simulink library "EngineModelsLibrary"  (R2014b)
settings: Solver=ode45  StartTime=0.0  StopTime=10.0  RelTol=1e-3
values from neighbouring files (symbols this model uses):
  k = 0.2    [ES_Run.m]    (also in ES_Run_v2.m = 10)
undefined symbols (not defined in the file or in its folder): b, COBRA_Compressor, cp, CPT_COBRA_LIB, D, etalim, gam, Newton, Pa, PARAM, Pl, pref, Ps, R, Raphson, rlim, T_0, Tref, Wclim
undefined symbols (not defined in the file): cr, e, etagain, fit_pars, kL, kS, par
(part 1 of 3)
settings Model: Creator=Mike  LastModifiedBy=rsalehi

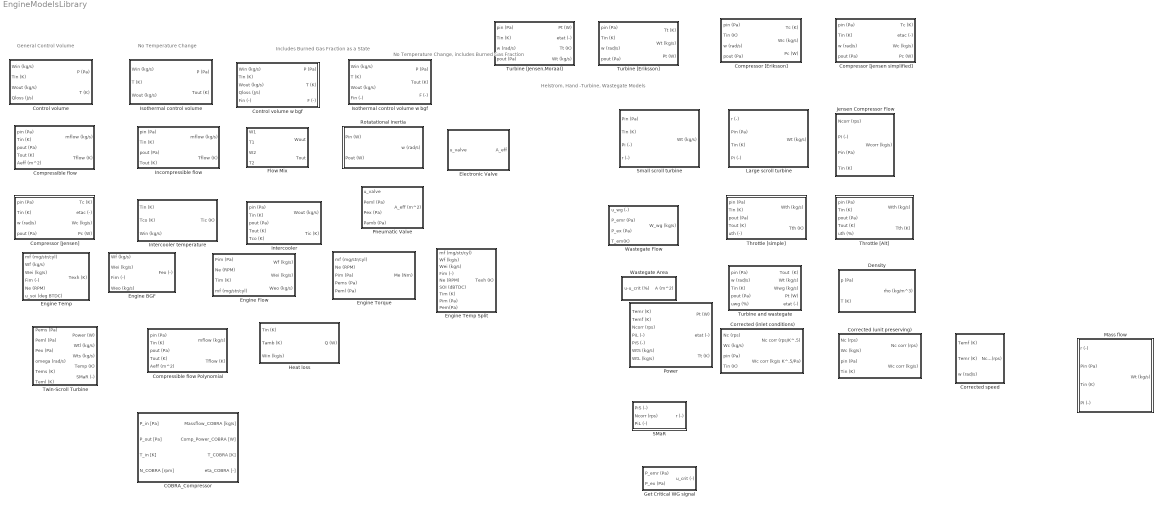
== system EngineModelsLibrary ==
  note: Helstrom, Hand -Turbine, Wastegate Models
  note: No Temperature Change, includes Burned Gas Fraction
  note: Includes Burned Gas Fraction as a State
  note: No Temperature Change
  note: General Control Volume
  COBRA_Compressor : Subsystem  Tag=Version 2 Compressor model with lookup option for efficiency  AncestorBlock=CPT_COBRA_LIB/COBRA_Compressor  mask(Controlled Power Technologies Ltd){CompWheel=C80}
      mask prompts: CompWheel "Compressor Wheel"
      mask help:
      | Basic model of COBRA electric supercharger compressor
      |
      | INPUTS:
      |
      | P_in - Gas pressure upstream of the compressor [Pa]
      | P_out - Gas pressure downstream of the compressor [Pa]
      | T_in - Gas temperature upstream of the compressor [K]
      | N_COBRA - Compressor rotational speed [rpm]
      |
      | OUTPUTS:
      |
      | Massflow_COBRA - Gas mass flow through the compressor [kg/s]
      | Comp_Power_COBRA - Power consumed by the compressor due to aerodynamic load [W]
      | T_COBRA - Gas temperature at compressor outlet [K]
      | eta_COBRA - Compressor efficiency [-]
      |
      | Use the menu selector below to choose either the C70 or C80 compressor wheels
      |
      | For further information click help or consult documentation
      mask init:
      | try 
      | load('COBRA_Compressor_Pars.mat');
      | 
      | Wheel=get_param(gcb,'CompWheel');
      | if strcmp(Wheel,'C70')==1
      |     COBRACompressor.mdotcMap=COBRACompressor.mdotcMapC70;
      |     COBRACompressor.EtaMap=COBRACompressor.EtaMapC70;
      |     COBRACompressor.max_mdotc=COBRACompressor.max_mdotc_C70;
      |     disp('C70 Wheel selected');
      | else
      |     COBRACompressor.mdotcMap=COBRACompressor.mdotcMapC80;
      |     COBRACompressor.EtaMap=COBRACompressor.EtaMapC80;
      |     COBRACompressor.max_mdotc=COBRACompressor.max_mdotc_C80;
      |     disp('C80 Wheel selected');
      | end
      | 
      | catch InitErr
      |     disp('ERROR: COBRA_Compressor_Pars.mat file must be located in same directory as model or in a directory on the Matlab path')
      | end
      mask Help:
      | COBRA Compressor Model
      | 
      | Model Description
      | 
      | The COBRA compressor model comprises a simplified lookup table implementation of the compressor maps. Taking inputs of upstream temperature and pressure, downstream pressure and compressor rotational speed, it will calculate the compressor mass airflow, required shaft power, outlet gas temperature and overall compressor isentropic efficiency. The model is designed to be used in mean value simulations and needs to be connected to plenums / volumes either side of it to function correctly.
      | 
      | Model requirements, installation and usage notes
      | 
      | The model has been created using MATLAB / Simulink Release 2014b. To use the model it should be dragged and dropped into another the Simulink model. The parameter file <COBRA_Compressor_Pars.mat> must be located in the current working directory or in a directory on the Matlab path, it is automatically loaded when the model initialises.
      | 
      | The model acts as a flow restriction element within a full simulation of the engine gas path, it requires volumes or plenums to be connected both directly upstream and downstream of it in order to provide the input and output conditions required to calculate the mass flow. The resultant mass flow must be connected both as flow into the downstream volume and flow out of the upstream volume.
      | 
      | Normally the COBRA system is used with a bypass which can be either active or passive, this has not been provided in this model but can easily be created, consult the documentation for further details.
      | 
      | No electrical or mechanical dynamics have been included in this model. For an approximation of transient response, a 1st order lag can be placed in front of the speed input to COBRA with a T90 time of approx. 300ms.
      | 
      | The option to use 2 different compressor sizes is built-in to the model. Either the C70 or C80 wheels can be chosen from a menu within the block mask, double click on the block to access this menu.
      mask TypeOptions CompWheel: C70 | C80
      mask Display:
      | mytext=get_param(gcb,'CompWheel');
      | disp(strcat(mytext,'\n'));
      | disp('Compressor');
      | %text(40,17,'Controlled Power');
      | %text(40,5,'Technologies Ltd');
  Compressible flow : Subsystem  mask{gam=1.27, R=286, PIlin=.99}
      mask prompts: gam "Specific heat ratio (-)"; R "Ideal gas constant (J/kg/K)"; PIlin "Linear segment minimum pressure ratio (-)"
      mask help: Compressible flow, see App. C in Heywood (1988). Modified by adding a linear segment for pressure ratios larger than the parameter PIlin. In this way, it is possible to avoid infinite derivative for pressure ratios close to one. -- erikhe@umich
  Compressible flow Polynomial : Subsystem  mask{gam=1.27, R=286, P=fit_pars.egr.psi}
      mask prompts: gam "Specific heat ratio (-)"; R "Ideal gas constant (J/kg/K)"; P "Psi Polynomail [3 pars]"
      mask help: Compressible flow, see App. C in Heywood (1988). Modified by adding a linear segment for pressure ratios larger than the parameter PIlin. In this way, it is possible to avoid infinite derivative for pressure ratios close to one. -- erikhe@umich
  Compressor [Eriksson] : Subsystem  mask{gam=PARAM.air.gamma, cp=PARAM.air.cp, R=PARAM.air.R, D=PARAM.compressor.D, a1=PARAM.compressor.a1, a2=PARAM.compressor.a2, pref=PARAM.compressor.pref, Tref=PARAM.compressor.Tref, Phimax=PARAM.compressor.Phimax, Ncorrmax=PARAM.compressor.Ncorrmax, etamax=PARAM.compressor.etamax, etamin=PARAM.compressor.etamin, Q=PARAM.compressor.Q}
      mask prompts: gam "Specific heat ratio (-)"; cp "Specific heat cp (J/kg/K)"; R "Ideal gas constant (J/kg/K)"; D "Compressor diameter (m)"; a1 "Mass flow fit 1"; a2 "Mass flow fit 2"; pref "Reference pressure (Pa)"; Tref "Reference temperature (K)"; Phimax "Efficiency fit Phimax (-)"; Ncorrmax "Efficiency fit Ncorrmax (rps)"; etamax "Efficiency max (-)"; etamin "Efficiency min (-)"; Q "Efficiency fit matrix"
  Compressor [Jensen simplified] : Subsystem  mask{gam=PARAM.air.gamma, R=PARAM.air.R, D=PARAM.compressor.D, k11=PARAM.compressor.k11, k12=PARAM.compressor.k12, k21=PARAM.compressor.k21, k22=PARAM.compressor.k22, k31=PARAM.compressor.k31, k32=PARAM.compressor.k32, Wcmax=PARAM.compressor.Wcmax, Wcmin=PARAM.compressor.Wcmin, pref=PARAM.compressor.pref, Tref=PARAM.compressor.Tref, a11=PARAM.compressor.a11, a12=PARAM.compressor.a12, a13=PARAM.compressor.a13, a21=PARAM.compressor.a21, a22=PARAM.compressor.a22, a23=PARAM.compressor.a23, a31=PARAM.compressor.a31, a32=PARAM.compressor.a32, a33=PARAM.compressor.a33, etamax=PARAM.compressor.etamax, etamin=PARAM.compressor.etamin}
      mask prompts: gam "Specific heat ratio (-)"; R "Gas constant (J/kg/K)"; D "Compressor diameter (m)"; k11 "Mass flow fit k11"; k12 "Mass flow fit k12"; k21 "Mass flow fit k21"; k22 "Mass flow fit k22"; k31 "Mass flow fit k31"; k32 "Mass flow fit k32"; Wcmax "Mass flow max (kg/s)"; Wcmin "Mass flow min (kg/s)"; pref "Reference pressure (Pa)"; Tref "Reference temperature (K)"; a11 "Efficiency fit a11"; a12 "Efficiency fit a12"; a13 "Efficiency fit a13"; a21 "Efficiency fit a21"; a22 "Efficiency fit a22"; a23 "Efficiency fit a23"; a31 "Efficiency fit a31"; a32 "Efficiency fit a32"; a33 "Efficiency fit a33"; etamax "Efficiency max (-)"; etamin "Efficiency min (-)"
  Compressor [Jensen] : Subsystem  mask{gam=PARAM.air.gamma, R=PARAM.air.R, D=PARAM.compressor.D, K=PARAM.compressor.flow, Wcorr_lims=PARAM.compressor.Wclim, Pref=PARAM.compressor.Pref, Tref=PARAM.compressor.Tref, A=PARAM.compressor.eta, eta_lims=PARAM.compressor.etalim}
      mask prompts: gam "Specific heat ratio (-)"; R "Gas constant (J/kg/K)"; D "Compressor diameter (m)"; K "Mass flow fit (9 par)"; Wcorr_lims "Mass flow (min,max) (kg/s)"; Pref "Reference pressure (Pa)"; Tref "Reference temperature (K)"; A "Efficiency fit (9 par)"; eta_lims "Efficiency (min,max) (-)"
  Control volume : Subsystem  mask{V=.05, R=287, gam=1.4, Tinit=290, Pinit=1.2e5}
      mask prompts: V "Volume (m^3)"; R "Ideal gas constant (J/kg/K)"; gam "Specific heat ratio (-)"; Tinit "Initial temperature (K)"; Pinit "Initial pressure (Pa)"
      mask help: Thermodynamic control volume based on ideal mixing of perfect gases, see Ch, 14 in Heywood (1988) -- erikhe@umich.edu
  Control volume w bgf : Subsystem  mask{V=.05, R=287, gam=1.4, Tinit=300, Pinit=1.1e5, Finit=.2}
      mask prompts: V "Volume (m^3)"; R "Ideal gas constant (J/kg/K)"; gam "Specific heat ratio (-)"; Tinit "Initial temperature (K)"; Pinit "Initial pressure (Pa)"; Finit "Initial burned gas fraction (-)"
      mask help: Thermodynamic control volume based on ideal mixing of perfect gases, see Ch, 14 in Heywood (1988) -- erikhe@umich.edu
  Corrected (inlet conditions) : Subsystem
  Corrected (unit preserving) : Subsystem
  Corrected speed : Subsystem
  Density : Subsystem
  Electronic Valve : Subsystem  mask{A_fit=0}
      mask prompts: A_fit "Polynomial Fit Parameter [3 pars]"
  Engine BGF : Subsystem  mask{AFs=14.5}
      mask prompts: AFs "Stoichiometric Air-Fuel Ratio (-)"
  Engine Flow : Subsystem  mask{R=0, ncyl=0, VD=0, c_etav=0}
      mask prompts: R "Cylinder gas constant (J/kgK)"; ncyl "Num. Cylinders (-)"; VD "Displacement volume (m^3)"; c_etav "Volumetric efficiency fit parameters [5 pars]"
  Engine Temp : Subsystem  mask{c_Tex=e.CylinderParams.Tex, Te_lim=e.CylinderParams.Texlim}
      mask prompts: c_Tex "Cylinder Temp Pars [5 pars]"; Te_lim "Exhaust Temp Limits (K) [min max]"
  "Engine Temp Split " : Subsystem  mask{c_Tex=e.CylinderParams.Tex, Te_lim=e.CylinderParams.Texlim, gam=0}
      mask prompts: c_Tex "Cylinder Temp Pars [5 pars]"; Te_lim "Exhaust Temp Limits (K) [min max]"; gam "Cylinder ratio of specific heats (-)"
  Engine Torque : Subsystem  mask{ncyl=0, VD=0, qlhv=0, CR=0, gam=0, eta_c=0, fric_c=0}
      mask prompts: ncyl "Num. Cylinders (-)"; VD "Displacement volume (m^3)"; qlhv "Lower Heating Value (J/kg)"; CR "Compression Ratio (-)"; gam "Ratio of Specific Heats"; eta_c "Combustion efficiency (-)"; fric_c "Engine Friction [3 pars]"
  Flow Mix : Subsystem  mask{cp_s=0}
      mask prompts: cp_s "Flow cps (J/(kgK) [cp1 cp2]"
  Get Critical WG signal : Subsystem
  Heat loss : Subsystem  mask{Q_fit=PARAM.intercooler.a0}
      mask prompts: Q_fit "Q fit [3 pars]"
  Incompressible flow : Subsystem  mask{C=0, P_lin=0}
      mask prompts: C "Flow resistance ()"; P_lin "Linear segment maximum pressure loss (Pa)"
      mask help: Compressible flow for turbulent flow, see e.g. Eriksson et.al. (2002) Modeling and simulation of a turbo charged SI engine, Annual Reviews in Control. Modified by adding a linear segment for pressure losses smaller than the parameter dPlin. In this way, it is possible to avoid infinite derivative for pressure losses close to zero. -- erikhe@umich
  Intercooler : Subsystem  mask{a0=PARAM.intercooler.a0, a1=PARAM.intercooler.a1, a2=PARAM.intercooler.a2, C=PARAM.intercooler.C, dPlin=PARAM.intercooler.dPlin}
      mask prompts: a0 "Efficiency fit a0 (-)"; a1 "Efficiency fit a1 (s/kg"; a2 "Efficiency fit a2 (1/K)"; C "Flow resistance ()"; dPlin "Linear segment maximum pressure loss (Pa)"
  Intercooler temperature : Subsystem  mask{a=PARAM.intercooler.a0}
      mask prompts: a "Efficiency fit [3 pars]"
  Isothermal control volume : Subsystem  mask{V=.02, R=287, Pinit=1.1e5}
      mask prompts: V "Volume (m^3)"; R "Ideal gas constant (J/kg/K)"; Pinit "Initial pressure (Pa)"
      mask help: Thermodynamic control volume based on ideal mixing of perfect gases, see Ch, 14 in Heywood (1988) -- erikhe@umich.edu
  Isothermal control volume w bgf : Subsystem  mask{V=.05, R=287, Pinit=1.1e5, Finit=.2}
      mask prompts: V "Volume (m^3)"; R "Ideal gas constant (J/kg/K)"; Pinit "Initial pressure (Pa)"; Finit "Initial burned gas fraction (-)"
      mask help: Thermodynamic control volume based on ideal mixing of perfect gases, see Ch, 14 in Heywood (1988) -- erikhe@umich.edu
  "Jensen Compressor Flow " : Subsystem
  Large scroll turbine : Subsystem  mask{gam=gam, cp=cp, D=D, k=kL, Wclim=Wclim}
      mask prompts: gam "Ratio of specific heats (-)"; cp "Specific heat cp (J/kg/K)"; D "Diameter (m)"; k "Mass flow fit (4 par)"; Wclim "Mass flow (min,max) (kg/s K^.5/Pa)"
  Mass flow : Subsystem
  Pneumatic Valve : Subsystem  mask{A_fit=e.TC.wg.Area_coeff, wg_Ps=e.TC.wg.Ps, wg_K=e.TC.wg.K, wg_Pl=e.TC.wg.Pl}
      mask prompts: A_fit "Area Fit Parameter (m^2)"; wg_Ps "Valve Spring Pressure (kPa)"; wg_K "Valve Fit Constant, K (-)"; wg_Pl "Valve Line Pressure (kPa)"
  Power : Subsystem  mask{gam=gam, cp=cp, D=D, Tref=Tref, b=b, gain=etagain, etalim=etalim}
      mask prompts: gam "gamma"; D "Diameter (m)"; b "Efficiency fit (7 par)"; gain "Efficiency gain (-)"; etalim "Efficiency (min,max) (-)"
  Rotatational inertia : Subsystem  mask{J=0, b=0, om_lims=0, om_init=0}
      mask prompts: J "Inertia (kg m^2)"; b "Friction coefficient (Nm s/rad)"; om_lims "Speed Limits (rad/s) [min max]"; om_init "Initial speed (rad/s)"
  SMaR : Subsystem  mask{c=cr, rlim=rlim}
      mask prompts: c "SMaR fit (8 par)"; rlim "SMaR (min,max) (-)"
  Small scroll turbine : Subsystem  mask{gam=gam, cp=cp, D=D, k=kS, Wclim=Wclim}
      mask prompts: gam "Ratio of specific heats (-)"; cp "Specific heat cp (J/kg/K)"; D "Diameter (m)"; k "Mass flow fit (4 par)"; Wclim "Mass flow (min,max) (kg/s K^.5/Pa)"
  Throttle [Alt] : Subsystem  mask{gam=PARAM.air.gamma, R=PARAM.air.R, PIlin=PARAM.throttle.PIlin, Ar0=PARAM.throttle.A0, Ar1=PARAM.throttle.A1, a0=PARAM.throttle.a0, a1=PARAM.throttle.a1, a2=PARAM.throttle.a2, b0=PARAM.throttle.b0, b1=PARAM.throttle.b1}
      mask prompts: gam "Specific heat ratio (-)"; R "Ideal gas constant (J/kg/K)"; PIlin "Linear segment minimum pressure ratio (-)"; Ar0 "Throttle parameter A0 (m^2)"; Ar1 "Throttle parameter A1 (m^2)"; a0 "Throttle parameter a0"; a1 "Throttle parameter a1"; a2 "Throttle parameter a2"; b0 "Throttle parameter b0"; b1 "Throttle parameter b1"
  Throttle [simple] : Subsystem  mask{gam=PARAM.air.gamma, R=PARAM.air.R, Amax=PARAM.throttle.Amax, Amin=PARAM.throttle.Amin, PIlin=PARAM.throttle.PIlin}
      mask prompts: gam "Specific heat ratio (-)"; R "Ideal gas constant (J/kg/K)"; Amax "Throttle max area (m^2)"; Amin "Throttle min area (m^2)"; PIlin "Linear segment minimum pressure ratio (-)"
  Turbine [Eriksson] : Subsystem  mask{gam=PARAM.exh.gamma, cp=PARAM.exh.cp, D=PARAM.turbine.D, k0=PARAM.turbine.k0, k1=PARAM.turbine.k1, ct=PARAM.turbine.ct, BSRmax=PARAM.turbine.BSRmax, etamax=PARAM.turbine.etamax, etamin=PARAM.turbine.etamin}
      mask prompts: gam "Ratio of specific heats (-)"; cp "Specific heat cp (J/kg/K)"; D "Diameter (m)"; k0 "Mass flow fit parameter k0"; k1 "Mass flow fit parameter k1"; ct "Efficiency fit parameter ct"; BSRmax "BSR max (-)"; etamax "Efficiency max (-)"; etamin "Efficiency min (-)"
  Turbine [Jensen,Moraal] : Subsystem  mask{gam=PARAM.exh.gamma, cp=PARAM.exh.cp, D=PARAM.turbine.D, k11=PARAM.turbine.k11, k12=PARAM.turbine.k12, k21=PARAM.turbine.k21, k22=PARAM.turbine.k22, PIlin=PARAM.turbine.PIlin, Wtcmax=PARAM.turbine.Wtcmax, Wtcmin=PARAM.turbine.Wtcmin, b0=PARAM.turbine.b0, b1=PARAM.turbine.b1, b2=PARAM.turbine.b2, b3=PARAM.turbine.b3, b4=PARAM.turbine.b4, b5=PARAM.turbine.b5, etamax=PARAM.turbine.etamax, etamin=PARAM.turbine.etamin}
      mask prompts: gam "Ratio of specific heats (-)"; cp "Specific heat cp (J/kg/K)"; D "Diameter (m)"; k11 "Mass flow fit k11"; k12 "Mass flow fit k12"; k21 "Mass flow fit k21"; k22 "Mass flow fit k22"; PIlin "Mass flow PIlin"; Wtcmax "Mass flow max (kg/s K^.5/Pa)"; Wtcmin "Mass flow min (kg/s K^.5/Pa)"; b0 "Efficiency fit b0"; b1 "Efficiency fit b1"; b2 "Efficiency fit b2"; b3 "Efficiency fit b3"; b4 "Efficiency fit b4"; b5 "Efficiency fit b5"; etamax "Efficiency max (-)"; etamin "Efficiency min (-)"
  Turbine and wastegate : Subsystem
  Twin-Scroll Turbine : Subsystem  mask{smar_fit=e.TC.turb.smar, smar_lim=e.TC.turb.smarlim, flow_fit=e.TC.turb.large.flow, flow_lim=e.TC.turb.Wclim, eta=e.TC.turb.etagain*.85, gam=e.Gases.ex.gamma, cp=e.Gases.ex.cp}
      mask prompts: smar_fit "SMaR Fit Pars [5 pars]"; smar_lim "SMaR Limits [min max]"; flow_fit "Large Scroll Flow Fit Pars [4 pars]"; flow_lim "Large Scroll Flow Limits [min max]"; eta "Turbine Efficiency (-)"; gam "Specific Heat Ratio (-)"; cp "Const. Pressure Specific Heat (J/kgK)"
  "Wastegate Area " : Subsystem  mask{c=par.tc.wg.Area_coeff}
      mask prompts: c "Area fit functions (4 params)"
  "Wastegate Flow " : Subsystem  mask{gam=gam, R=par.tc.wg.R, Pa=par.amb.P*1e-3, Pl=par.tc.wg.Pl, Ps=par.tc.wg.Ps, k=par.tc.wg.K}
      mask prompts: gam "Ratio of specific heats []"; R "Gas Constant [J/(kg*K]"; Pa "Atmospheric Pressure [kPa]"; Pl "Valve Line Pressure [kPa]"; Ps "Valve Opening Pressure [kPa]"; k "Valve Area Ratio []"

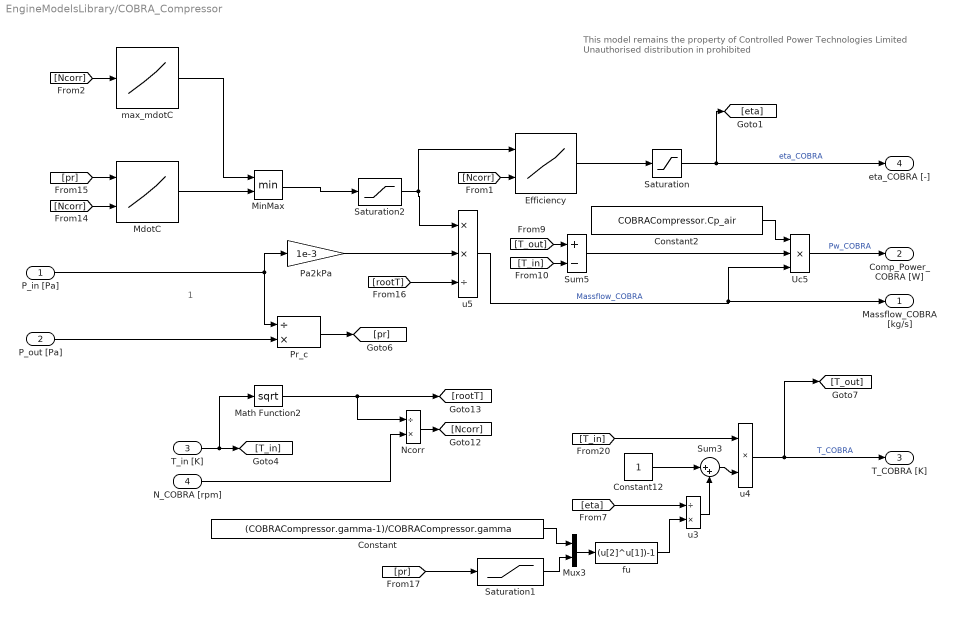
== system EngineModelsLibrary/COBRA_Compressor ==
  note: This model remains the property of Controlled Power Technologies Limited
      | Unauthorised distribution in prohibited
  note: 1
  P_in [Pa] : Inport
  P_out [Pa] : Inport  Port=2
  T_in [K] : Inport  Port=3
  N_COBRA [rpm] : Inport  Port=4
  Constant : Constant  Value=(COBRACompressor.gamma-1)/COBRACompressor.gamma
  Constant12 : Constant
  Constant2 : Constant  Value=COBRACompressor.Cp_air
  Efficiency : Lookup_n-D  BreakpointsForDimension1=COBRACompressor.EtaMap.y  BreakpointsForDimension2=COBRACompressor.EtaMap.x  Table=COBRACompressor.EtaMap.z  InternalRulePriority=Speed  RndMeth=Simplest  InputSameDT=on
  Math Function2 : Math  Operator=sqrt  SaturateOnIntegerOverflow=on
  MdotC : Lookup_n-D  BreakpointsForDimension1=COBRACompressor.mdotcMap.y  BreakpointsForDimension2=COBRACompressor.mdotcMap.x  Table=COBRACompressor.mdotcMap.z  InternalRulePriority=Speed  RndMeth=Simplest  InputSameDT=on
  MinMax : MinMax  Inputs=2
  Mux3 : Mux  Inputs=2
  Ncorr : Product  Inputs=/*  SaturateOnIntegerOverflow=on  RndMeth=Zero  InputSameDT=on  OutDataTypeStr=Inherit: Same as first input
  Pa2kPa : Gain  Gain=1e-3  SaturateOnIntegerOverflow=on  OutDataTypeStr=Inherit: Same as input  ParamDataTypeStr=Inherit: Same as input
  Pr_c : Product  Inputs=/*  SaturateOnIntegerOverflow=on  RndMeth=Zero  InputSameDT=on  OutDataTypeStr=Inherit: Same as first input
  Saturation : Saturate  UpperLimit=COBRACompressor.etac_max  LowerLimit=COBRACompressor.etac_min
  Saturation1 : Saturate  UpperLimit=Inf  LowerLimit=1
  Saturation2 : Saturate  UpperLimit=Inf  LowerLimit=0
  Sum3 : Sum  Inputs=|++  SaturateOnIntegerOverflow=on  InputSameDT=on  OutDataTypeStr=Inherit: Same as first input
  Sum5 : Sum  Inputs=+-  SaturateOnIntegerOverflow=on  InputSameDT=on  OutDataTypeStr=Inherit: Same as first input
  Uc5 : Product  Inputs=3  SaturateOnIntegerOverflow=on  RndMeth=Zero  InputSameDT=on  OutDataTypeStr=Inherit: Same as first input
  fu : Fcn  Expr=(u[2]^u[1])-1
  max_mdotC : Lookup_n-D  NumberOfTableDimensions=1  BreakpointsForDimension1=COBRACompressor.max_mdotc.y  Table=COBRACompressor.max_mdotc.x  InternalRulePriority=Speed  RndMeth=Simplest  InputSameDT=on
  u3 : Product  Inputs=/*  SaturateOnIntegerOverflow=on  RndMeth=Zero  InputSameDT=on  OutDataTypeStr=Inherit: Same as first input
  u4 : Product  SaturateOnIntegerOverflow=on  RndMeth=Zero  InputSameDT=on  OutDataTypeStr=Inherit: Same as first input
  u5 : Product  Inputs=**/  SaturateOnIntegerOverflow=on  RndMeth=Zero  InputSameDT=on  OutDataTypeStr=Inherit: Same as first input
  Massflow_COBRA [kg/s] : Outport  InitialOutput=T_0
  Comp_Power_COBRA [W] : Outport  Port=2  InitialOutput=T_0
  T_COBRA [K] : Outport  Port=3  InitialOutput=T_0
  eta_COBRA [-] : Outport  Port=4  InitialOutput=T_0
  wires:
  Mux3/1 -> fu/1
  Constant/1 -> Mux3/1
  Saturation1/1 -> Mux3/2
  [pr] -> Saturation1/1
  [eta] -> u3/1
  u4/1 -> T_COBRA [K]/1, [T_out]  "T_COBRA"
  Sum3/1 -> u4/2
  Constant12/1 -> Sum3/1
  u3/1 -> Sum3/2
  [T_in] -> u4/1
  fu/1 -> u3/2
  Pr_c/1 -> [pr]
  Math Function2/1 -> [rootT], Ncorr/1
  N_COBRA [rpm]/1 -> Ncorr/2
  Ncorr/1 -> [Ncorr]
  P_out [Pa]/1 -> Pr_c/2
  T_in [K]/1 -> [T_in], Math Function2/1
  Pa2kPa/1 -> u5/2
  Saturation/1 -> [eta], eta_COBRA [-]/1  "eta_COBRA"
  Uc5/1 -> Comp_Power_COBRA [W]/1  "Pw_COBRA"
  Sum5/1 -> Uc5/2
  u5/1 -> Uc5/3, Massflow_COBRA [kg/s]/1  "Massflow_COBRA"
  [rootT] -> u5/3
  Efficiency/1 -> Saturation/1
  [pr] -> MdotC/1
  [T_in] -> Sum5/2
  [Ncorr] -> Efficiency/2
  Constant2/1 -> Uc5/1
  [T_out] -> Sum5/1
  [Ncorr] -> MdotC/2
  P_in [Pa]/1 -> Pa2kPa/1, Pr_c/1
  Saturation2/1 -> Efficiency/1, u5/1
  [Ncorr] -> max_mdotC/1
  max_mdotC/1 -> MinMax/1
  MdotC/1 -> MinMax/2
  MinMax/1 -> Saturation2/1

== system EngineModelsLibrary/Compressible flow ==
  note: Compressible flow, see App. C in Heywood (1988). Modified by adding a linear segment for pressure ratios larger than
      | the parameter PIlin. In this way, it is possible to avoid infinite derivative for pressure ratios close to one. -- erikhe@umich
  pin (Pa) : Inport
  Tin (K) : Inport  Port=2
  pout (Pa) : Inport  Port=3
  Tout (K) : Inport  Port=4
  Aeff (m^2) : Inport  Port=5
  Demux : Demux  Outputs=2
  Mux : Mux  Inputs=5
  S-Function : S-Function  FunctionName=compressible_flow  Parameters=R,gam,PIlin  SFunctionModules=compressible_flow engine_model  EnableBusSupport=off
  mflow (kg/s) : Outport
  Tflow (K) : Outport  Port=2
  wires:
  Demux/1 -> mflow (kg/s)/1
  pin (Pa)/1 -> Mux/1
  Tin (K)/1 -> Mux/2
  pout (Pa)/1 -> Mux/3
  Mux/1 -> S-Function/1
  S-Function/1 -> Demux/1
  Demux/2 -> Tflow (K)/1
  Tout (K)/1 -> Mux/4
  Aeff (m^2)/1 -> Mux/5

== system EngineModelsLibrary/Compressible flow Polynomial ==
  note: Compressible flow, see App. C in Heywood (1988). Modified by adding a linear segment for pressure ratios larger than
      | the parameter PIlin. In this way, it is possible to avoid infinite derivative for pressure ratios close to one. -- erikhe@umich
  pin (Pa) : Inport
  Tin (K) : Inport  Port=2
  pout (Pa) : Inport  Port=3
  Tout (K) : Inport  Port=4
  Aeff (m^2) : Inport  Port=5
  Demux : Demux  Outputs=2
  Mux : Mux  Inputs=5
  S-Function : S-Function  FunctionName=compressible_flow_poly  Parameters=R,gam,P  SFunctionModules=compressible_flow_poly engine_model  EnableBusSupport=off
  mflow (kg/s) : Outport
  Tflow (K) : Outport  Port=2
  wires:
  Demux/1 -> mflow (kg/s)/1
  pin (Pa)/1 -> Mux/1
  Tin (K)/1 -> Mux/2
  pout (Pa)/1 -> Mux/3
  Mux/1 -> S-Function/1
  S-Function/1 -> Demux/1
  Demux/2 -> Tflow (K)/1
  Tout (K)/1 -> Mux/4
  Aeff (m^2)/1 -> Mux/5

== system EngineModelsLibrary/Compressor [Eriksson] ==
  pin (Pa) : Inport
  Tin (K) : Inport  Port=2
  w (rad/s) : Inport  Port=3
  pout (Pa) : Inport  Port=4
  Corrected flow inv (unit preserving) : Subsystem
  Corrected speed : Subsystem
  Density : Subsystem
  Efficiency : Subsystem
  Mass flow : Subsystem
  Power : Subsystem
  Pressure ratio : Subsystem
  Temperature : Subsystem
  To Workspace2 : ToWorkspace  VariableName=etac  SampleTime=-1
  Tc (K) : Outport
  Wc (kg/s) : Outport  Port=2
  Pc (W) : Outport  Port=3
  wires:
  Corrected flow inv (unit preserving)/1(W (kg/s)) -> Wc (kg/s)/1, Power/1(W (kg/s))
  pout (Pa)/1 -> Pressure ratio/2(pout (Pa))
  pin (Pa)/1 -> Corrected flow inv (unit preserving)/2(pin (Pa)), Density/1(p (Pa)), Mass flow/3(pin (Pa)), Pressure ratio/1(pin (Pa))
  w (rad/s)/1 -> Corrected speed/1(w (rad/s))
  Pressure ratio/1(PI (-)) -> Temperature/2(PI (-)), Mass flow/2(PI (-))
  Corrected speed/1(Ncorr (rps)) -> Mass flow/1(Ncorr (rps)), Efficiency/3(Ncorr (rps))
  Density/1(rho (kg/m^3)) -> Efficiency/2(rho (kg/m^3))
  Tin (K)/1 -> Corrected flow inv (unit preserving)/3(Tin (K)), Density/2(T (K)), Corrected speed/2(Tin (K)), Mass flow/4(Tin (K)), Temperature/1(Tin (K)), Power/2(Tin (K))
  Mass flow/1(Wcorr (kg/s)) -> Corrected flow inv (unit preserving)/1(Wcorr (kg/s)), Efficiency/1(Wcorr (kg/s))
  Efficiency/1(etac (-)) -> To Workspace2/1, Temperature/3(etac (-))
  Temperature/1(Tout (K)) -> Power/3(Tout (K)), Tc (K)/1
  Power/1(P (W)) -> Pc (W)/1

== system EngineModelsLibrary/Compressor [Jensen simplified] ==
  pin (Pa) : Inport
  Tin (K) : Inport  Port=2
  w (rad/s) : Inport  Port=3
  pout (Pa) : Inport  Port=4
  Corrected flow inv (unit preserving) : Subsystem
  Corrected speed : Subsystem
  Density : Subsystem
  Efficiency : Subsystem
  Mass flow : Subsystem
  Power : Subsystem
  Pressure ratio : Subsystem
  Temperature : Subsystem
  Tc (K) : Outport
  etac (-) : Outport  Port=2
  Wc (kg/s) : Outport  Port=3
  Pc (W) : Outport  Port=4
  wires:
  Power/1(P (W)) -> Pc (W)/1
  Temperature/1(Tout (K)) -> Tc (K)/1, Power/3(Tout (K))
  Efficiency/1(etac (-)) -> Temperature/3(etac (-)), etac (-)/1
  Mass flow/1(Wcorr (kg/s)) -> Efficiency/1(Wcorr (kg/s)), Corrected flow inv (unit preserving)/1(Wcorr (kg/s))
  Tin (K)/1 -> Power/2(Tin (K)), Temperature/1(Tin (K)), Efficiency/4(Tin (K)), Mass flow/4(Tin (K)), Corrected speed/2(Tin (K)), Density/2(T (K)), Corrected flow inv (unit preserving)/3(Tin (K))
  Density/1(rho (kg/m^3)) -> Efficiency/2(rho (kg/m^3))
  Corrected speed/1(Ncorr (rps)) -> Efficiency/3(Ncorr (rps)), Mass flow/1(Ncorr (rps))
  Pressure ratio/1(PI (-)) -> Mass flow/2(PI (-)), Temperature/2(PI (-))
  w (rad/s)/1 -> Corrected speed/1(w (rad/s))
  pin (Pa)/1 -> Pressure ratio/1(pin (Pa)), Mass flow/3(pin (Pa)), Density/1(p (Pa)), Corrected flow inv (unit preserving)/2(pin (Pa))
  pout (Pa)/1 -> Pressure ratio/2(pout (Pa))
  Corrected flow inv (unit preserving)/1(W (kg/s)) -> Power/1(W (kg/s)), Wc (kg/s)/1

== system EngineModelsLibrary/Compressor [Jensen] ==
  pin (Pa) : Inport
  Tin (K) : Inport  Port=2
  w (rad/s) : Inport  Port=3
  pout (Pa) : Inport  Port=4
  Demux : Demux
  Mux : Mux
  S-Function : S-Function  FunctionName=compressor  Parameters=R, gam, D,K,A,Tref,Pref,Wcorr_lims,eta_lims  SFunctionModules=compressor engine_model  EnableBusSupport=off
  Tc (K) : Outport
  etac (-) : Outport  Port=2
  Wc (kg/s) : Outport  Port=3
  Pc (W) : Outport  Port=4
  wires:
  Demux/1 -> Tc (K)/1
  pin (Pa)/1 -> Mux/1
  Tin (K)/1 -> Mux/2
  w (rad/s)/1 -> Mux/3
  Mux/1 -> S-Function/1
  S-Function/1 -> Demux/1
  Demux/2 -> etac (-)/1
  pout (Pa)/1 -> Mux/4
  Demux/4 -> Pc (W)/1
  Demux/3 -> Wc (kg/s)/1

== system EngineModelsLibrary/Control volume ==
  note: Thermodynamic control volume based on ideal mixing of perfect gases, see Ch, 14 in Heywood (1988) -- erikhe@umich.edu
  Win (kg/s) : Inport
  Tin (K) : Inport  Port=2
  Wout (kg/s) : Inport  Port=3
  Qloss (J/s) : Inport  Port=4
  Demux : Demux  Outputs=2
  Mux : Mux
  S-Function : S-Function  FunctionName=control_volume  Parameters=V,R,gam,Pinit,Tinit  SFunctionModules=control_volume engine_model  EnableBusSupport=off
  P (Pa) : Outport
  T (K) : Outport  Port=2
  wires:
  Demux/1 -> P (Pa)/1
  Win (kg/s)/1 -> Mux/1
  Tin (K)/1 -> Mux/2
  Wout (kg/s)/1 -> Mux/3
  Qloss (J/s)/1 -> Mux/4
  Mux/1 -> S-Function/1
  S-Function/1 -> Demux/1
  Demux/2 -> T (K)/1

== system EngineModelsLibrary/Control volume w bgf ==
  note: Thermodynamic control volume based on ideal mixing of perfect gases, see Ch, 14 in Heywood (1988) -- erikhe@umich.edu
  Win (kg/s) : Inport
  Tin (K) : Inport  Port=2
  Wout (kg/s) : Inport  Port=3
  Qloss (J/s) : Inport  Port=4
  Fin (-) : Inport  Port=5
  Demux : Demux  Outputs=3
  Mux : Mux  Inputs=5
  S-Function : S-Function  FunctionName=bgf_control_volume  Parameters=V,R,gam,Pinit,Tinit,Finit  SFunctionModules=bgf_control_volume engine_model  EnableBusSupport=off
  P (Pa) : Outport
  T (K) : Outport  Port=2
  F (-) : Outport  Port=3
  wires:
  Demux/1 -> P (Pa)/1
  Win (kg/s)/1 -> Mux/1
  Tin (K)/1 -> Mux/2
  Wout (kg/s)/1 -> Mux/3
  Qloss (J/s)/1 -> Mux/4
  Mux/1 -> S-Function/1
  S-Function/1 -> Demux/1
  Demux/2 -> T (K)/1
  Fin (-)/1 -> Mux/5
  Demux/3 -> F (-)/1

== system EngineModelsLibrary/Corrected (inlet conditions) ==
  note: Speed and mass flow corrected based on inlet conditions.
      | -- erikhe@umich
  Nc (rps) : Inport
  Wc (kg/s) : Inport  Port=2
  pin (Pa) : Inport  Port=3
  Tin (K) : Inport  Port=4
  Divide1 : Product  Inputs=*/
  Divide3 : Product  Inputs=**/
  Math Function : Math  Operator=sqrt  SaturateOnIntegerOverflow=on
  Nc corr (rps/K^.5) : Outport
  Wc corr (kg/s K^.5/Pa) : Outport  Port=2
  wires:
  pin (Pa)/1 -> Divide3/3
  Tin (K)/1 -> Math Function/1
  Nc (rps)/1 -> Divide1/1
  Math Function/1 -> Divide1/2, Divide3/1
  Divide1/1 -> Nc corr (rps/K^.5)/1
  Wc (kg/s)/1 -> Divide3/2
  Divide3/1 -> Wc corr (kg/s K^.5/Pa)/1

== system EngineModelsLibrary/Corrected (unit preserving) ==
  note: Speed and mass flow corrected based on inlet conditions and reference state.
      | -- erikhe@umich
  Nc (rps) : Inport
  Wc (kg/s) : Inport  Port=2
  pin (Pa) : Inport  Port=3
  Tin (K) : Inport  Port=4
  Constant : Constant  Value=Tref
  Constant2 : Constant  Value=pref
  Divide : Product  Inputs=*/
  Divide1 : Product  Inputs=*/
  Divide2 : Product  Inputs=*/
  Divide3 : Product  Inputs=**/
  Math Function : Math  Operator=sqrt  SaturateOnIntegerOverflow=on
  Nc corr (rps) : Outport
  Wc corr (kg/s) : Outport  Port=2
  wires:
  Divide3/1 -> Wc corr (kg/s)/1
  Wc (kg/s)/1 -> Divide3/2
  Divide2/1 -> Divide3/3
  pin (Pa)/1 -> Divide2/1
  Constant2/1 -> Divide2/2
  Divide1/1 -> Nc corr (rps)/1
  Math Function/1 -> Divide3/1, Divide1/2
  Nc (rps)/1 -> Divide1/1
  Tin (K)/1 -> Divide/1
  Constant/1 -> Divide/2
  Divide/1 -> Math Function/1

== system EngineModelsLibrary/Corrected speed ==
  note: Speed corrected based on inlet conditions and reference state.
      | -- erikhe@umich
  Temf (K) : Inport
  Temr (K) : Inport  Port=2
  w (rad/s) : Inport  Port=3
  Constant : Constant  Value=Tref
  Divide : Product  Inputs=*/
  Divide1 : Product  Inputs=*/
  Gain : Gain  Gain=.5
  Gain1 : Gain  Gain=1/(2*pi)
  Math Function : Math  Operator=sqrt  SaturateOnIntegerOverflow=on
  Sum : Sum  Inputs=|++
  Ncorr (rps) : Outport
  wires:
  Gain1/1 -> Divide1/1
  Divide1/1 -> Ncorr (rps)/1
  Math Function/1 -> Divide1/2
  Constant/1 -> Divide/2
  Divide/1 -> Math Function/1
  w (rad/s)/1 -> Gain1/1
  Sum/1 -> Gain/1
  Temf (K)/1 -> Sum/1
  Gain/1 -> Divide/1
  Temr (K)/1 -> Sum/2

== system EngineModelsLibrary/Density ==
  p (Pa) : Inport
  T (K) : Inport  Port=2
  Constant1 : Constant  Value=R
  Product : Product  Inputs=*//  RndMeth=Zero
  rho (kg/m^3) : Outport
  wires:
  Product/1 -> rho (kg/m^3)/1
  Constant1/1 -> Product/3
  T (K)/1 -> Product/2
  p (Pa)/1 -> Product/1

== system EngineModelsLibrary/Electronic Valve ==
  "u_valve " : Inport
  S-Function : S-Function  FunctionName=electronic_valve  Parameters=A_fit  SFunctionModules=electronic_valve engine_model  EnableBusSupport=off
  A_eff : Outport
  wires:
  "u_valve "/1 -> S-Function/1
  S-Function/1 -> A_eff/1

== system EngineModelsLibrary/Engine BGF ==
  Wf (kg/s) : Inport
  Wei (kg/s) : Inport  Port=2
  Fim (-) : Inport  Port=3
  Weo (kg/s) : Inport  Port=4
  Mux2 : Mux
  S-Function : S-Function  FunctionName=engine_bgf  Parameters=AFs  SFunctionModules=engine_bgf engine_model  EnableBusSupport=off
  Feo (-) : Outport
  wires:
  Mux2/1 -> S-Function/1
  S-Function/1 -> Feo (-)/1
  Wei (kg/s)/1 -> Mux2/2
  Fim (-)/1 -> Mux2/3
  Weo (kg/s)/1 -> Mux2/4
  Wf (kg/s)/1 -> Mux2/1

== system EngineModelsLibrary/Engine Flow ==
  Pim (Pa) : Inport
  Ne (RPM) : Inport  Port=2
  Tim (K) : Inport  Port=3
  mf (mg/str/cyl) : Inport  Port=4
  Demux : Demux  Outputs=3
  Mux2 : Mux
  S-Function : S-Function  FunctionName=engine_flow  Parameters=R,ncyl,VD,c_etav  SFunctionModules=engine_flow engine_model  EnableBusSupport=off
  Wf (kg/s) : Outport
  Wei (kg/s) : Outport  Port=2
  Weo (kg/s) : Outport  Port=3
  wires:
  Pim (Pa)/1 -> Mux2/1
  Ne (RPM)/1 -> Mux2/2
  Tim (K)/1 -> Mux2/3
  Mux2/1 -> S-Function/1
  mf (mg/str/cyl)/1 -> Mux2/4
  Demux/1 -> Wf (kg/s)/1
  S-Function/1 -> Demux/1
  Demux/2 -> Wei (kg/s)/1
  Demux/3 -> Weo (kg/s)/1

== system EngineModelsLibrary/Engine Temp ==
  mf (mg/str/cyl) : Inport
  Wf (kg/s) : Inport  Port=2
  Wei (kg/s) : Inport  Port=3
  Fim (-) : Inport  Port=4
  Ne (RPM) : Inport  Port=5
  u_soi (deg BTDC) : Inport  Port=6
  Mux2 : Mux  Inputs=6
  S-Function : S-Function  FunctionName=engine_temp  Parameters=c_Tex, Te_lim  SFunctionModules=engine_temp engine_model  EnableBusSupport=off
  Texh (K) : Outport
  wires:
  Mux2/1 -> S-Function/1
  mf (mg/str/cyl)/1 -> Mux2/1
  S-Function/1 -> Texh (K)/1
  Wei (kg/s)/1 -> Mux2/3
  Fim (-)/1 -> Mux2/4
  Ne (RPM)/1 -> Mux2/5
  Wf (kg/s)/1 -> Mux2/2
  u_soi (deg BTDC)/1 -> Mux2/6

== system EngineModelsLibrary/Engine Temp Split  ==
  mf (mg/str/cyl) : Inport
  Wf (kg/s) : Inport  Port=2
  Wei (kg/s) : Inport  Port=3
  Fim (-) : Inport  Port=4
  Ne (RPM) : Inport  Port=5
  SOI (dBTDC) : Inport  Port=6
  Tim (K) : Inport  Port=7
  Pim (Pa) : Inport  Port=8
  Pem(Pa) : Inport  Port=9
  Mux2 : Mux  Inputs=9
  S-Function : S-Function  FunctionName=engine_temp_split  Parameters=c_Tex, Te_lim,gam  SFunctionModules=engine_temp_split engine_model  EnableBusSupport=off
  Texh (K) : Outport
  wires:
  Mux2/1 -> S-Function/1
  mf (mg/str/cyl)/1 -> Mux2/1
  S-Function/1 -> Texh (K)/1
  Wei (kg/s)/1 -> Mux2/3
  Fim (-)/1 -> Mux2/4
  Ne (RPM)/1 -> Mux2/5
  Wf (kg/s)/1 -> Mux2/2
  Tim (K)/1 -> Mux2/7
  SOI (dBTDC)/1 -> Mux2/6
  Pim (Pa)/1 -> Mux2/8
  Pem(Pa)/1 -> Mux2/9

== system EngineModelsLibrary/Engine Torque ==
  mf (mg/str/cyl) : Inport
  Ne (RPM) : Inport  Port=2
  Pim (Pa) : Inport  Port=3
  Pems (Pa) : Inport  Port=4
  Peml (Pa) : Inport  Port=5
  Mux2 : Mux  Inputs=5
  S-Function : S-Function  FunctionName=engine_torque  Parameters=ncyl,qlhv,CR,gam,eta_c,VD,fric_c  SFunctionModules=engine_torque engine_model  EnableBusSupport=off
  Me (Nm) : Outport
  wires:
  Mux2/1 -> S-Function/1
  mf (mg/str/cyl)/1 -> Mux2/1
  S-Function/1 -> Me (Nm)/1
  Pim (Pa)/1 -> Mux2/3
  Pems (Pa)/1 -> Mux2/4
  Peml (Pa)/1 -> Mux2/5
  Ne (RPM)/1 -> Mux2/2

== system EngineModelsLibrary/Flow Mix ==
  "W1 " : Inport
  T1 : Inport  Port=2
  W2 : Inport  Port=3
  "T2 " : Inport  Port=4
  Demux1 : Demux  Outputs=2
  Mux : Mux
  S-Function : S-Function  FunctionName=flow_mix  Parameters=cp_s  SFunctionModules=flow_mix engine_model  EnableBusSupport=off
  Wout : Outport
  "Tout " : Outport  Port=2
  wires:
  Mux/1 -> S-Function/1
  "W1 "/1 -> Mux/1
  T1/1 -> Mux/2
  W2/1 -> Mux/3
  "T2 "/1 -> Mux/4
  Demux1/1 -> Wout/1
  S-Function/1 -> Demux1/1
  Demux1/2 -> "Tout "/1

== system EngineModelsLibrary/Get Critical WG signal ==
  P_emr (Pa) : Inport
  P_ex (Pa) : Inport  Port=2
  Add : Sum  Inputs=+-+
  Add1 : Sum
  Constant : Constant  Value=Ps
  Constant1 : Constant  Value=k
  Constant2 : Constant  Value=Pa
  Constant3 : Constant  Value=Pl
  Divide : Product  Inputs=*/
  Divide1 : Product  Inputs=*/
  Gain : Gain  Gain=1e-3
  Gain1 : Gain  Gain=1e-3
  u_crit (-) : Outport
  wires:
  Gain1/1 -> Add/2
  Gain/1 -> Add/3
  Divide1/1 -> u_crit (-)/1
  Constant3/1 -> Divide1/2
  Add1/1 -> Divide1/1
  Constant2/1 -> Add1/2
  Divide/1 -> Add1/1
  Constant1/1 -> Divide/2
  Add/1 -> Divide/1
  Constant/1 -> Add/1
  P_ex (Pa)/1 -> Gain/1
  P_emr (Pa)/1 -> Gain1/1

== system EngineModelsLibrary/Heat loss ==
  note: Manifold Heat Loss
  Tin (K) : Inport
  Tamb (K) : Inport  Port=2
  Win (kg/s) : Inport  Port=3
  Mux : Mux  Inputs=2
  S-Function : S-Function  FunctionName=manifold_heat_loss  Parameters=Q_fit  SFunctionModules=manifold_heat_loss engine_model  EnableBusSupport=off
  Sum : Sum  Inputs=|+-
  Q (W) : Outport
  wires:
  S-Function/1 -> Q (W)/1
  Tin (K)/1 -> Sum/1
  Tamb (K)/1 -> Sum/2
  Win (kg/s)/1 -> Mux/2
  Mux/1 -> S-Function/1
  Sum/1 -> Mux/1

== system EngineModelsLibrary/Incompressible flow ==
  note: Incompressible flow , see e.g. Eriksson et.al. (2002) Modeling and simulation of a turbo charged SI engine,
      | Annual Reviews in Control. Modified by adding a linear segment for pressure losses smaller than the parameter dPlin.
      | In this way, it is possible to avoid infinite derivative for pressure losses close to zero. -- erikhe@umich
  pin (Pa) : Inport
  Tin (K) : Inport  Port=2
  pout (Pa) : Inport  Port=3
  Tout (K) : Inport  Port=4
  Demux1 : Demux  Outputs=2
  Mux2 : Mux
  S-Function : S-Function  FunctionName=incompressible_flow  Parameters=P_lin,C  SFunctionModules=incompressible_flow engine_model  EnableBusSupport=off
  mflow (kg/s) : Outport
  Tflow (K) : Outport  Port=2
  wires:
  Demux1/1 -> mflow (kg/s)/1
  pin (Pa)/1 -> Mux2/1
  Tin (K)/1 -> Mux2/2
  pout (Pa)/1 -> Mux2/3
  Mux2/1 -> S-Function/1
  S-Function/1 -> Demux1/1
  Demux1/2 -> Tflow (K)/1
  Tout (K)/1 -> Mux2/4

== system EngineModelsLibrary/Intercooler ==
  pin (Pa) : Inport
  Tin (K) : Inport  Port=2
  pout (Pa) : Inport  Port=3
  Tout (K) : Inport  Port=4
  Tco (K) : Inport  Port=5
  Intercooler flow resistance : Subsystem  mask{C=C, dPlin=dPlin}
      mask prompts: C "Flow resistance ()"; dPlin "Linear segment maximum pressure loss (Pa)"
      mask help: Compressible flow for turbulent flow, see e.g. Eriksson et.al. (2002) Modeling and simulation of a turbo charged SI engine, Annual Reviews in Control. Modified by adding a linear segment for pressure losses smaller than the parameter dPlin. In this way, it is possible to avoid infinite derivative for pressure losses close to zero. -- erikhe@umich
  Intercooler temperature : Subsystem  mask{a0=PARAM.intercooler.a0, a1=PARAM.intercooler.a1, a2=PARAM.intercooler.a2}
      mask prompts: a0 "Efficiency fit a0 (-)"; a1 "Efficiency fit a1 (s/kg)"; a2 "Efficiency fit a2 (1/K)"
  Wout (kg/s) : Outport
  Tic (K) : Outport  Port=2
  wires:
  Intercooler temperature/1(Tic (K)) -> Tic (K)/1
  Tout (K)/1 -> Intercooler flow resistance/4(Tout (K))
  pout (Pa)/1 -> Intercooler flow resistance/3(pout (Pa))
  Tin (K)/1 -> Intercooler flow resistance/2(Tin (K))
  pin (Pa)/1 -> Intercooler flow resistance/1(pin (Pa))
  Intercooler flow resistance/2(Tflow (K)) -> Intercooler temperature/3(Tin (K))
  Intercooler flow resistance/1(mflow (kg/s)) -> Intercooler temperature/2(Win (kg/s)), Wout (kg/s)/1
  Tco (K)/1 -> Intercooler temperature/1(Tco (K))

== system EngineModelsLibrary/Intercooler temperature ==
  note: Intercooler temperature model, see e.g. Eriksson et al. (2002)
      | Modeling of a turbocharged SI engine, Annual reviews in Control.
      | -- erikhe@umich
  Tin (K) : Inport
  Tco (K) : Inport  Port=2
  Win (kg/s) : Inport  Port=3
  Mux : Mux  Inputs=3
  S-Function : S-Function  FunctionName=cooler_temp  Parameters=a  SFunctionModules=cooler_temp engine_model  EnableBusSupport=off
  Tic (K) : Outport
  wires:
  S-Function/1 -> Tic (K)/1
  Tin (K)/1 -> Mux/1
  Tco (K)/1 -> Mux/2
  Win (kg/s)/1 -> Mux/3
  Mux/1 -> S-Function/1

== system EngineModelsLibrary/Isothermal control volume ==
  note: Thermodynamic control volume based on ideal mixing of perfect gases, see Ch, 14 in Heywood (1988) -- erikhe@umich.edu
  Win (kg/s) : Inport
  T (K) : Inport  Port=2
  Wout (kg/s) : Inport  Port=3
  Mux : Mux  Inputs=3
  S-Function : S-Function  FunctionName=iso_control_volume  Parameters=V,R,Pinit  SFunctionModules=iso_control_volume engine_model  EnableBusSupport=off
  P (Pa) : Outport
  Tout (K) : Outport  Port=2
  wires:
  Win (kg/s)/1 -> Mux/1
  Wout (kg/s)/1 -> Mux/2
  Mux/1 -> S-Function/1
  T (K)/1 -> Tout (K)/1, Mux/3
  S-Function/1 -> P (Pa)/1

== system EngineModelsLibrary/Isothermal control volume w bgf ==
  note: Thermodynamic control volume based on ideal mixing of perfect gases, see Ch, 14 in Heywood (1988) -- erikhe@umich.edu
  Win (kg/s) : Inport
  T (K) : Inport  Port=2
  Wout (kg/s) : Inport  Port=3
  Fin (-) : Inport  Port=4
  Demux : Demux  Outputs=2
  Mux : Mux
  S-Function1 : S-Function  FunctionName=iso_bgf_control_volume  Parameters=V,R,Pinit,Finit  SFunctionModules=iso_bgf_control_volume engine_model  EnableBusSupport=off
  P (Pa) : Outport
  Tout (K) : Outport  Port=2
  F (-) : Outport  Port=3
  wires:
  Demux/1 -> P (Pa)/1
  Win (kg/s)/1 -> Mux/1
  Wout (kg/s)/1 -> Mux/2
  Fin (-)/1 -> Mux/3
  Demux/2 -> F (-)/1
  S-Function1/1 -> Demux/1
  Mux/1 -> S-Function1/1
  T (K)/1 -> Tout (K)/1, Mux/4

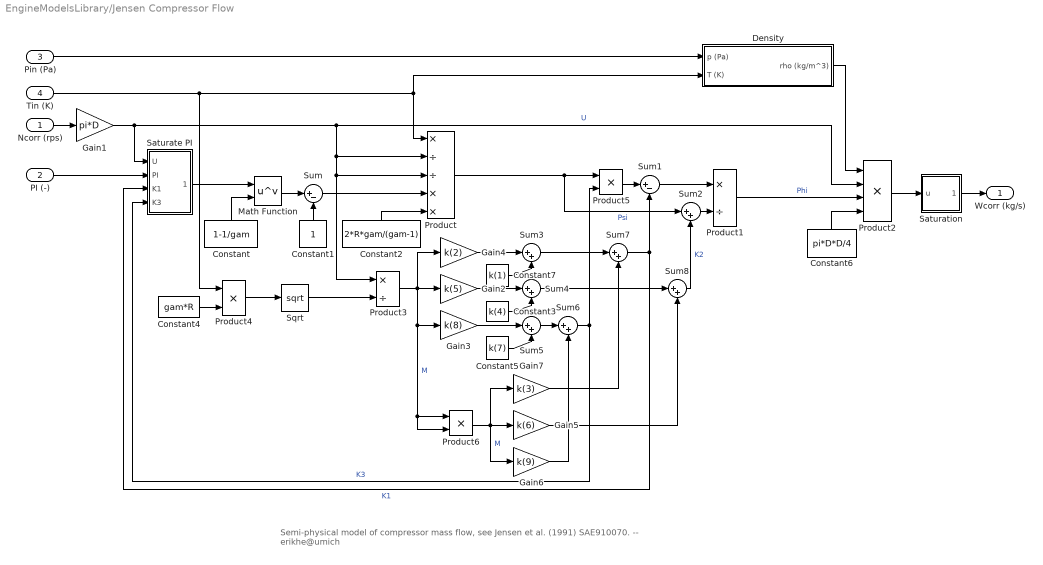
== system EngineModelsLibrary/Jensen Compressor Flow  ==
  note: Semi-physical model of compressor mass flow, see Jensen et al. (1991) SAE910070.
      | -- erikhe@umich
  Ncorr (rps) : Inport
  PI (-) : Inport  Port=2
  Pin (Pa) : Inport  Port=3
  Tin (K) : Inport  Port=4
  Constant : Constant  Value=1-1/gam
  Constant1 : Constant
  Constant2 : Constant  Value=2*R*gam/(gam-1)
  Constant3 : Constant  Value=k(4)
  Constant4 : Constant  Value=gam*R
  Constant5 : Constant  Value=k(7)
  Constant6 : Constant  Value=pi*D*D/4
  Constant7 : Constant  Value=k(1)
  Density : Subsystem
  Gain1 : Gain  Gain=pi*D
  Gain2 : Gain  Gain=k(5)
  Gain3 : Gain  Gain=k(8)
  Gain4 : Gain  Gain=k(2)
  Gain5 : Gain  Gain=k(6)
  Gain6 : Gain  Gain=k(9)
  Gain7 : Gain  Gain=k(3)
  Math Function : Math  Operator=pow  SaturateOnIntegerOverflow=on
  Product : Product  Inputs=*//**  RndMeth=Zero
  Product1 : Product  Inputs=*/  RndMeth=Zero
  Product2 : Product  Inputs=4  RndMeth=Zero
  Product3 : Product  Inputs=*/  RndMeth=Zero
  Product4 : Product  RndMeth=Zero
  Product5 : Product  RndMeth=Zero
  Product6 : Product  RndMeth=Zero
  Saturate PI : Subsystem
  Saturation : Subsystem  mask{lim=Wclim}
      mask prompts: lim "Saturation limits (min,max)"
  Sqrt : Sqrt  AlgorithmType=Newton-Raphson  SaturateOnIntegerOverflow=on
  Sum : Sum  Inputs=|+-
  Sum1 : Sum  Inputs=|+-
  Sum{2..8} (7 alike) : Sum  Inputs=|++
  Wcorr (kg/s) : Outport
  wires:
  Product5/1 -> Sum1/1
  Constant5/1 -> Sum5/2
  Constant3/1 -> Sum4/2
  Constant7/1 -> Sum3/2
  Gain3/1 -> Sum5/1
  Gain2/1 -> Sum4/1
  Gain4/1 -> Sum3/1
  Product3/1 -> Gain4/1, Gain2/1, Gain3/1, Product6/1, Product6/2  "M"
  Constant4/1 -> Product4/2
  Product4/1 -> Sqrt/1
  Sqrt/1 -> Product3/2
  Gain1/1 -> Saturate PI/1(U), Product2/2, Product3/1, Product/3, Product/2  "U"
  Sum2/1 -> Product1/2
  Sum1/1 -> Product1/1
  Density/1(rho (kg/m^3)) -> Product2/1
  Product2/1 -> Saturation/1(u)
  Constant6/1 -> Product2/4
  Product1/1 -> Product2/3  "Phi"
  Product/1 -> Product5/1, Sum2/1  "Psi"
  Constant2/1 -> Product/5
  Sum/1 -> Product/4
  Ncorr (rps)/1 -> Gain1/1
  Constant1/1 -> Sum/2
  Math Function/1 -> Sum/1
  Constant/1 -> Math Function/2
  Tin (K)/1 -> Product4/1, Product/1, Density/2(T (K))
  Pin (Pa)/1 -> Density/1(p (Pa))
  Saturation/1(Sat(u)) -> Wcorr (kg/s)/1
  Sum5/1 -> Sum6/1
  Sum6/1 -> Saturate PI/4(K3), Product5/2  "K3"
  Sum3/1 -> Sum7/1
  Sum7/1 -> Saturate PI/3(K1), Sum1/2  "K1"
  Sum4/1 -> Sum8/1
  Sum8/1 -> Sum2/2  "K2"
  Product6/1 -> Gain6/1, Gain7/1, Gain5/1  "M"
  Gain7/1 -> Sum7/2
  Gain5/1 -> Sum8/2
  Gain6/1 -> Sum6/2
  Saturate PI/1(PIsat) -> Math Function/1
  PI (-)/1 -> Saturate PI/2(PI)

== system EngineModelsLibrary/Large scroll turbine ==
  r (-) : Inport
  Pin (Pa) : Inport  Port=2
  Tin (K) : Inport  Port=3
  Pi (-) : Inport  Port=4
  Mass flow : Subsystem
  Wt (kg/s) : Outport
  wires:
  r (-)/1 -> Mass flow/1(r (-))
  Mass flow/1(Wt (kg/s)) -> Wt (kg/s)/1
  Pi (-)/1 -> Mass flow/4(PI (-))
  Pin (Pa)/1 -> Mass flow/2(Pin (Pa))
  Tin (K)/1 -> Mass flow/3(Tin (K))

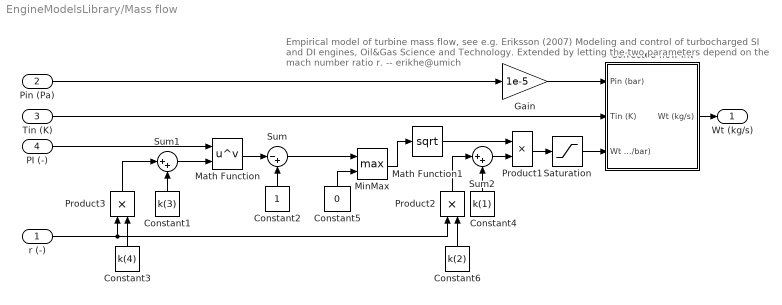
== system EngineModelsLibrary/Mass flow ==
  note: Empirical model of turbine mass flow, see e.g. Eriksson (2007)
      | Modeling and control of turbocharged SI and DI engines, Oil&Gas Science and Technology.
      | Extended by letting the two parameters depend on the mach number ratio r.
      | -- erikhe@umich
  r (-) : Inport
  Pin (Pa) : Inport  Port=2
  Tin (K) : Inport  Port=3
  PI (-) : Inport  Port=4
  Constant1 : Constant  Value=k(3)
  Constant2 : Constant
  Constant3 : Constant  Value=k(4)
  Constant4 : Constant  Value=k(1)
  Constant5 : Constant  Value=0
  Constant6 : Constant  Value=k(2)
  Corrected flow inv : Subsystem
  Gain : Gain  Gain=1e-5
  Math Function : Math  Operator=pow  SaturateOnIntegerOverflow=on
  Math Function1 : Math  Operator=sqrt  SaturateOnIntegerOverflow=on
  MinMax : MinMax  Function=max  Inputs=2
  Product1 : Product  RndMeth=Zero
  Product2 : Product  RndMeth=Zero
  Product3 : Product  RndMeth=Zero
  Saturation : Saturate  UpperLimit=Wclim(2)  LowerLimit=Wclim(1)
  Sum : Sum  Inputs=|-+
  Sum1 : Sum  Inputs=|++
  Sum2 : Sum  Inputs=|++
  Wt (kg/s) : Outport
  wires:
  Saturation/1 -> Corrected flow inv/3(Wt corr (kg/s K^.5/bar))
  Gain/1 -> Corrected flow inv/1(Pin (bar))
  Constant6/1 -> Product2/2
  Product2/1 -> Sum2/1
  Constant4/1 -> Sum2/2
  Sum2/1 -> Product1/2
  r (-)/1 -> Product2/1, Product3/1
  Constant3/1 -> Product3/2
  Product3/1 -> Sum1/1
  Constant1/1 -> Sum1/2
  Sum1/1 -> Math Function/2
  Corrected flow inv/1(Wt (kg/s)) -> Wt (kg/s)/1
  Sum/1 -> MinMax/1
  MinMax/1 -> Math Function1/1
  Constant5/1 -> MinMax/2
  PI (-)/1 -> Math Function/1
  Math Function/1 -> Sum/1
  Constant2/1 -> Sum/2
  Pin (Pa)/1 -> Gain/1
  Tin (K)/1 -> Corrected flow inv/2(Tin (K))
  Math Function1/1 -> Product1/1
  Product1/1 -> Saturation/1

== system EngineModelsLibrary/Pneumatic Valve ==
  "u_valve " : Inport
  Peml (Pa) : Inport  Port=2
  Pex (Pa) : Inport  Port=3
  Pamb (Pa) : Inport  Port=4
  Mux2 : Mux
  S-Function : S-Function  FunctionName=pneumatic_valve  Parameters=A_fit, wg_Ps, wg_K, wg_Pl  SFunctionModules=pneumatic_valve engine_model  EnableBusSupport=off
  A_eff (m^2) : Outport
  wires:
  S-Function/1 -> A_eff (m^2)/1
  Mux2/1 -> S-Function/1
  Peml (Pa)/1 -> Mux2/2
  Pex (Pa)/1 -> Mux2/3
  Pamb (Pa)/1 -> Mux2/4
  "u_valve "/1 -> Mux2/1

== system EngineModelsLibrary/Power ==
  Temr (K) : Inport
  Temf (K) : Inport  Port=2
  Ncorr (rps) : Inport  Port=3
  PiL (-) : Inport  Port=4
  PiS (-) : Inport  Port=5
  WtS (kg/s) : Inport  Port=6
  WtL (kg/s) : Inport  Port=7
  Efficiency : Subsystem
  Gain1 : Gain  Gain=.5
  Gain2 : Gain  Gain=.5
  Power : Subsystem
  Sum : Sum  Inputs=|++
  Sum1 : Sum  Inputs=|++
  Sum2 : Sum  Inputs=++|
  Temperature : Subsystem
  Pt (W) : Outport
  etat (-) : Outport  Port=2
  Tt (K) : Outport  Port=3
  wires:
  Efficiency/1(etat (-)) -> Temperature/3(etat (-)), etat (-)/1
  Temperature/1(Tout (K)) -> Tt (K)/1, Power/3(Tout (K))
  Sum/1 -> Gain1/1
  Temf (K)/1 -> Sum/1
  Temr (K)/1 -> Sum/2
  Gain1/1 -> Power/2(Tin (K)), Temperature/2(Tin (K))
  Sum1/1 -> Gain2/1
  PiL (-)/1 -> Sum1/2
  PiS (-)/1 -> Sum1/1
  Gain2/1 -> Efficiency/1(PI (-)), Temperature/1(PI (-))
  Ncorr (rps)/1 -> Efficiency/2(Ncorr (rps))
  Power/1(P (W)) -> Pt (W)/1
  Sum2/1 -> Power/1(W (kg/s))
  WtL (kg/s)/1 -> Sum2/2
  WtS (kg/s)/1 -> Sum2/1

== system EngineModelsLibrary/Rotatational inertia ==
  Pin (W) : Inport
  Pout (W) : Inport  Port=2
  Mux : Mux  Inputs=2
  S-Function : S-Function  FunctionName=rotational_inertia  Parameters=J,b,om_lims,om_init  SFunctionModules=rotational_inertia omega_init  EnableBusSupport=off
  w (rad/s) : Outport
  wires:
  Pin (W)/1 -> Mux/1
  Pout (W)/1 -> Mux/2
  Mux/1 -> S-Function/1
  S-Function/1 -> w (rad/s)/1

== system EngineModelsLibrary/SMaR ==
  PiS (-) : Inport
  Ncorr (rps) : Inport  Port=2
  PiL (-) : Inport  Port=3
  Constant : Constant  Value=c(1)
  Constant1 : Constant  Value=c(5)
  Gain : Gain  Gain=c(2)
  Gain1 : Gain  Gain=c(3)
  Gain2 : Gain  Gain=c(6)
  Gain3 : Gain  Gain=c(7)
  Gain4 : Gain  Gain=c(4)
  Gain5 : Gain  Gain=c(8)
  Product : Product  RndMeth=Zero
  Product1 : Product  RndMeth=Zero
  Saturation : Saturate  UpperLimit=rlim(2)  LowerLimit=rlim(1)
  Sum : Sum  Inputs=+++
  Sum1 : Sum  Inputs=+++
  Sum2 : Sum  Inputs=+++
  Sum3 : Sum  Inputs=|++
  r (-) : Outport
  wires:
  Constant/1 -> Sum/1
  Gain/1 -> Sum/2
  Gain1/1 -> Sum/3
  PiS (-)/1 -> Gain/1, Product1/1, Gain2/1
  PiL (-)/1 -> Gain1/1, Product1/2, Gain3/1
  Ncorr (rps)/1 -> Product/2
  Sum2/1 -> Saturation/1
  Product1/1 -> Gain4/1, Gain5/1
  Product/1 -> Sum2/3
  Sum/1 -> Sum2/1
  Gain4/1 -> Sum2/2
  Saturation/1 -> r (-)/1
  Constant1/1 -> Sum1/1
  Gain2/1 -> Sum1/2
  Gain3/1 -> Sum1/3
  Gain5/1 -> Sum3/2
  Sum3/1 -> Product/1
  Sum1/1 -> Sum3/1

== system EngineModelsLibrary/Small scroll turbine ==
  Pin (Pa) : Inport
  Tin (K) : Inport  Port=2
  Pi (-) : Inport  Port=3
  r (-) : Inport  Port=4
  Mass flow : Subsystem
  Wt (kg/s) : Outport
  wires:
  Tin (K)/1 -> Mass flow/3(Tin (K))
  Pin (Pa)/1 -> Mass flow/2(Pin (Pa))
  Pi (-)/1 -> Mass flow/4(PI (-))
  Mass flow/1(Wt (kg/s)) -> Wt (kg/s)/1
  r (-)/1 -> Mass flow/1(r (-))
